simulink model "topic2_2"  (R2019b)
settings: Solver=VariableStepAuto  StartTime=0.0  StopTime=0.12  RelTol=1e-3
libraries: powerlib x15, powerlib_meascontrol x9
settings Model: Creator=dell  LastModifiedBy=96547
settings DataIOCC: ReturnWorkspaceOutputs=off
settings DebuggingCC: ArithmeticOperatorsInVariantConditions=warning
settings SFSimCC: CustomCodeUndefinedFunction=UseInterfaceOnly

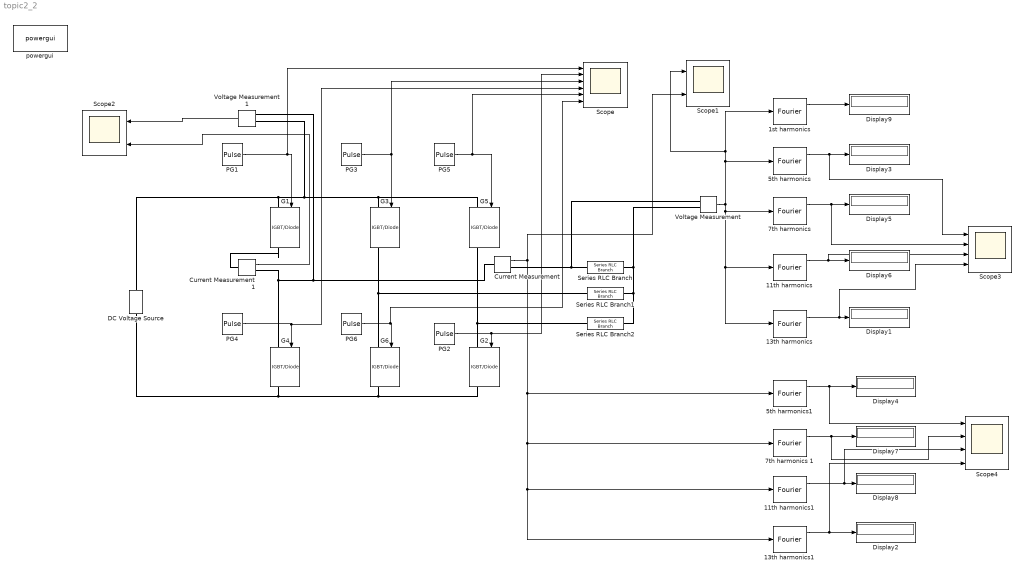
== system topic2_2 ==
  "  7th harmonics " : powerlib_meascontrol/Measurements/Fourier  Freq=50  n=7  InInit=[0, 0]  Ts=0
      settings: SourceProductName=Simscape Electrical
  "  7th harmonics 1" : powerlib_meascontrol/Measurements/Fourier  Freq=50  n=7  InInit=[0, 0]  Ts=0
      settings: SourceProductName=Simscape Electrical
  " 11th harmonics" : powerlib_meascontrol/Measurements/Fourier  Freq=50  n=11  InInit=[0, 0]  Ts=0
      settings: SourceProductName=Simscape Electrical
  " 11th harmonics1" : powerlib_meascontrol/Measurements/Fourier  Freq=50  n=11  InInit=[0, 0]  Ts=0
      settings: SourceProductName=Simscape Electrical
  " 13th harmonics" : powerlib_meascontrol/Measurements/Fourier  Freq=50  n=13  InInit=[0, 0]  Ts=0
      settings: SourceProductName=Simscape Electrical
  " 13th harmonics1" : powerlib_meascontrol/Measurements/Fourier  Freq=50  n=13  InInit=[0, 0]  Ts=0
      settings: SourceProductName=Simscape Electrical
  1st harmonics : powerlib_meascontrol/Measurements/Fourier  Freq=50  n=1  InInit=[0, 0]  Ts=0
      settings: SourceProductName=Simscape Electrical
  5th harmonics : powerlib_meascontrol/Measurements/Fourier  Freq=50  n=5  InInit=[0, 0]  Ts=0
      settings: SourceProductName=Simscape Electrical
  5th harmonics1 : powerlib_meascontrol/Measurements/Fourier  Freq=50  n=5  InInit=[0, 0]  Ts=0
      settings: SourceProductName=Simscape Electrical
  Current Measurement : powerlib/Measurements/Current Measurement  PhasorSimulation=off  OutputType=Complex  PSBequivalent=0
      settings: SourceProductName=Simscape Electrical
  Current Measurement1 : powerlib/Measurements/Current Measurement  PhasorSimulation=off  OutputType=Complex  PSBequivalent=0
      settings: SourceProductName=Simscape Electrical
  DC Voltage Source : powerlib/Electrical Sources/DC Voltage Source  Amplitude=200  Measurements=None
      settings: SourceProductName=Simscape Electrical
  Display{1..9} (9 alike) : Display
  G{1..6} (6 alike) : powerlib/Power Electronics/IGBT//Diode  Ron=1e-3  Rs=1e5  Cs=inf  Measurements=on
      settings: SourceProductName=Simscape Electrical
  PG1 : DiscretePulseGenerator  PulseType=Time based  Period=0.02  PulseWidth=50
  PG2 : DiscretePulseGenerator  PulseType=Time based  Period=0.02  PulseWidth=50  PhaseDelay=0.02*(2/3)+0.01
  PG3 : DiscretePulseGenerator  PulseType=Time based  Period=0.02  PulseWidth=50  PhaseDelay=0.02*(1/3)
  PG4 : DiscretePulseGenerator  PulseType=Time based  Period=0.02  PulseWidth=50  PhaseDelay=0.01
  PG5 : DiscretePulseGenerator  PulseType=Time based  Period=0.02  PulseWidth=50  PhaseDelay=0.02*(2/3)
  PG6 : DiscretePulseGenerator  PulseType=Time based  Period=0.02  PulseWidth=50  PhaseDelay=0.02*(1/3)+0.01
  Scope : Scope  NumInputPorts=6
  Scope1 : Scope  NumInputPorts=2
  Scope2 : Scope  NumInputPorts=2
  Scope3 : Scope  NumInputPorts=4
  Scope4 : Scope  NumInputPorts=4
  Series RLC Branch : powerlib/Elements/Series RLC Branch  LConnTagsString=__new0  RConnTagsString=__new0  BranchType=RL  Resistance=5  Inductance=10e-3  SetiL0=off  InitialCurrent=0  Capacitance=1e-6  Setx0=off  InitialVoltage=0  Measurements=None
      settings: SourceProductName=Simscape Electrical
  Series RLC Branch1 : powerlib/Elements/Series RLC Branch  LConnTagsString=__new0  RConnTagsString=__new0  BranchType=RL  Resistance=5  Inductance=10e-3  SetiL0=off  InitialCurrent=0  Capacitance=1e-6  Setx0=off  InitialVoltage=0  Measurements=None
      settings: SourceProductName=Simscape Electrical
  Series RLC Branch2 : powerlib/Elements/Series RLC Branch  LConnTagsString=__new0  RConnTagsString=__new0  BranchType=RL  Resistance=5  Inductance=10e-3  SetiL0=off  InitialCurrent=0  Capacitance=1e-6  Setx0=off  InitialVoltage=0  Measurements=None
      settings: SourceProductName=Simscape Electrical
  Voltage Measurement : powerlib/Measurements/Voltage Measurement  PhasorSimulation=off  OutputType=Complex  PSBequivalent=0
      settings: SourceProductName=Simscape Electrical
  Voltage Measurement1 : powerlib/Measurements/Voltage Measurement  PhasorSimulation=off  OutputType=Complex  PSBequivalent=0
      settings: SourceProductName=Simscape Electrical
  powergui : powerlib/powergui  Priority=1  SimulationMode=Continuous  SampleTime=50e-6  frequency=60  Iterations=50  frequencyindice=0  Pbase=100e6  ErrMax=1e-4  UnitsV=kV  UnitsW=MW  buscounter=0  FunctionMessages=off  echomessages=off  EnableUseOfTLC=off  CurrentSourceSwitches=off  DisableSnubberDevices=off  DisableRonSwitches=off  DisableVfSwitches=off  DisplayEquations=off  AutomaticDiscreteSolvers=off  SolverType=Tustin/Backward Euler (TBE)  Interpol=off  ExternalGateDelay=off  methode=off  Ts=100  x0status=blocks  SPID=on  SwTol=0  HookPort=off  NonlinearTolerance=1e-4  nMaxIteration=100  ContinueOnMaxIteration=off  RestoreLinks=warning  ResistiveCurrentMeasurement=off  Frange=[0:2:500]  Ylog=off  Xlog=on  ShowGrid=off  save=off  variable=ZData  structure=0  ZoomFFT=off  StartTime=0.0  cycles=1  DisplayStyle=1  fundamental=60  FreqAxis=off  MaxFrequency=1000  frequencyindicesteady=1  RmsSteady=1  display=off
      settings: SourceProductName=Simscape Electrical
  wires:
  PG1/1 -> Scope/1, G1/1
  PG2/1 -> G2/1, Scope/2
  PG3/1 -> G3/1, Scope/3
  PG4/1 -> Scope/4, G4/1
  PG5/1 -> Scope/5, G5/1
  PG6/1 -> Scope/6, G6/1
  " 11th harmonics"/1 -> Scope3/3, Display6/1
  5th harmonics/1 -> Scope3/1, Display3/1
  "  7th harmonics "/1 -> Scope3/2, Display5/1
  Voltage Measurement/1 -> " 13th harmonics"/1, " 11th harmonics"/1, "  7th harmonics "/1, 1st harmonics/1, Scope1/1, 5th harmonics/1
  " 13th harmonics"/1 -> Scope3/4, Display1/1
  "  7th harmonics 1"/1 -> Scope4/2, Display7/1
  Current Measurement/1 -> " 13th harmonics1"/1, " 11th harmonics1"/1, "  7th harmonics 1"/1, 5th harmonics1/1, Scope1/2
  " 11th harmonics1"/1 -> Scope4/3, Display8/1
  Voltage Measurement1/1 -> Scope2/1
  Current Measurement1/1 -> Scope2/2
  5th harmonics1/1 -> Scope4/1, Display4/1
  " 13th harmonics1"/1 -> Scope4/4, Display2/1
  1st harmonics/1 -> Display9/1
  connections:
  Current Measurement/LConn1 -- Voltage Measurement1/LConn2 -- G4/LConn1 -- Current Measurement1/RConn1
  DC Voltage Source/RConn1 -- Voltage Measurement1/LConn1 -- G5/LConn1 -- G3/LConn1 -- G1/LConn1
  G3/RConn1 -- Series RLC Branch1/LConn1 -- G6/LConn1
  G5/RConn1 -- Series RLC Branch2/LConn1 -- G2/LConn1
  DC Voltage Source/LConn1 -- G2/RConn1 -- G6/RConn1 -- G4/RConn1
  Series RLC Branch/RConn1 -- Series RLC Branch2/RConn1 -- Series RLC Branch1/RConn1 -- Voltage Measurement/LConn2
  G1/RConn1 -- Current Measurement1/LConn1
  Voltage Measurement/LConn1 -- Series RLC Branch/LConn1 -- Current Measurement/RConn1
